simulink model "disturbed"  (R2023a)
settings: Solver=ode45  StartTime=0.0  StopTime=6000  RelTol=1e-8  AbsTol=1e-8
values from neighbouring files (symbols this model uses):
  I = diag(nominal.moi)    [disturbanceCaller.m]    (also in disturbanceODEcaller.m)
  nominal =     [MOInominal.mat]    (also in disturbanceCaller.m = rmfield(nominal,"name"))
  params =     [params.mat]
  X0 = [w0;E0;eps0;eta0;r0;v0]    [disturbanceCaller.m]    (also in disturbanceODEcaller.m)
settings Model: Creator=Josh2  LastModifiedBy=Josh2
settings ModelReferenceCC: EnableRefExpFcnMdlSchedulingChecks=on

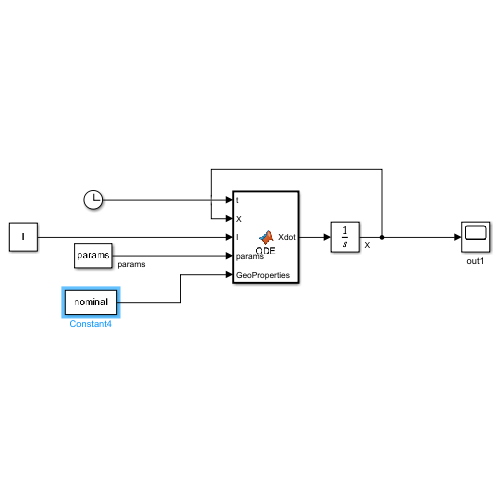
[thumbnail: Simulink's stored preview of the top-level diagram]
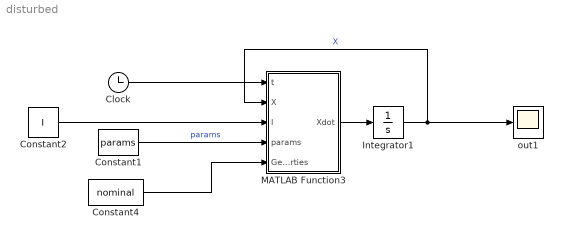
== system disturbed ==
  Clock : Clock
  Constant1 : Constant  Value=params  OutDataTypeStr=Bus: struggle
  Constant2 : Constant  Value=I
  Constant4 : Constant  Value=nominal  OutDataTypeStr=Bus: geoBus
  Integrator1 : Integrator  InitialCondition=X0
  MATLAB Function3 : MATLAB Function  TreatAsAtomicUnit=on
  out1 : Scope
  wires:
  Integrator1/1 -> out1/1, MATLAB Function3/2(X)  "X"
  Clock/1 -> MATLAB Function3/1(t)
  Constant1/1 -> MATLAB Function3/4(params)  "params"
  Constant2/1 -> MATLAB Function3/3(I)
  Constant4/1 -> MATLAB Function3/5(GeoProperties)
  MATLAB Function3/1(Xdot) -> Integrator1/1

== matlab function disturbed/MATLAB Function3 ==
  data: t input; Xdot output; X input; I input; params input; GeoProperties input
function Xdot = ODE(t,X,I,params,GeoProperties)



Xdot = SC_ODE(t,X,I,params,GeoProperties);
end
